simulink model "M_RALT"  (R2022a)
settings: Solver=ode4  StartTime=0.0  StopTime=100  FixedStep=0.01  RelTol=1e-3
PreLoadFcn:
  | listing = dir;
  | if (contains([listing .name], 'RALT')) && (contains([listing .name], 'MAP'))
  |     addpath('./RALT', './MAP', './DYN');
  |     addpath( genpath('./MAP') );
  | elseif (contains([listing .name], 'M_RALT.slx'))
  |     addpath('../RALT', '../MAP', '../DYN');
  |     addpath( genpath('../MAP') );
  | else
  | 
  | end
  | 
  | load('BUS_STRUCTURE_RALT.mat');
  | load('BUS_STRUCTURE_DYN.mat');
InitFcn:
  | listing = dir;
  | if (contains([listing .name], 'RALT')) && (contains([listing .name], 'MAP'))
  |     addpath('./RALT', './MAP', './DYN');
  |     addpath( genpath('./MAP') );
  | elseif (contains([listing .name], 'M_RALT.slx'))
  |     addpath('../RALT', '../MAP', '../DYN');
  |     addpath( genpath('../MAP') );
  | else
  | 
  | end
  | 
  | load('BUS_STRUCTURE_RALT.mat');
  | load('BUS_STRUCTURE_DYN.mat');
  | 
  | % Random number seed
  | if ~exist('ranNumSeed', 'var')
  |     ranNumSeed = 2034;
  | end
libraries: simulink x3
settings Model: Creator=ASCL  LastModifiedBy=ASCL
settings DataIOCC: SaveOutput=off  SignalLogging=off  DSMLogging=off  SaveTime=off  ReturnWorkspaceOutputs=off
settings OptimizationCC: BlockReduction=off  DefaultParameterBehavior=Inlined  UseDivisionForNetSlopeComputation=on  GainParamInheritBuiltInType=on  UseFloatMulNetSlope=on  ExpressionFolding=off  PassReuseOutputArgsAs=Individual arguments  ZeroExternalMemoryAtStartup=off  ZeroInternalMemoryAtStartup=off  EfficientFloat2IntCast=on  LifeSpan=inf  OptimizeBlockOrder=speed  DifferentSizesBufferReuse=on  EfficientTunableParamExpr=on
settings DebuggingCC: SignalInfNanChecking=warning  ReadBeforeWriteMsg=EnableAllAsError  WriteAfterWriteMsg=EnableAllAsError  WriteAfterReadMsg=EnableAllAsError  IntegerOverflowMsg=error  ParameterTunabilityLossMsg=error  UniqueDataStoreMsg=error  AssertControl=DisableAll  NonBusSignalsTreatedAsBus=error  SFInvalidInputDataAccessInChartInitDiag=error  SFTransitionOutsideNaturalParentDiag=error  SFUnreachableExecutionPathDiag=error  SFUndirectedBroadcastEventsDiag=error  IntegerSaturationMsg=error
settings HardwareCC: ProdBitPerPointer=32  ProdBitPerSizeT=32  ProdBitPerPtrDiffT=32  ProdLargestAtomicInteger=Long  ProdLargestAtomicFloat=Double  ProdEndianess=BigEndian  ProdWordSize=32  ProdLongLongMode=on  ProdHWDeviceType=Freescale->MPC83xx
settings ModelReferenceCC: ModelReferenceNumInstancesAllowed=Single
settings SFSimCC: SimCustomHeaderCode="#include \"MAP.h\""  SimUserSources=MAP.c  SimUserLibraries=WS2_32.LIB  CompileTimeRecursionLimit=0  EnableRuntimeRecursion=off  MATLABDynamicMemAlloc=off
settings RTWCC: SystemTargetFile=ert.tlc  TemplateMakefile=ert_default_tmf  GenerateReport=on  RTWUseSimCustomCode=on  CustomHeaderCode="#include \"MAP.h\""  CustomSource=MAP.c  CustomLibrary=WS2_32.LIB  BuildConfiguration=Faster Runs  IncludeHyperlinkInReport=on  LaunchReport=on  GenerateTraceInfo=on  GenerateTraceReport=on  GenerateTraceReportSl=on  GenerateTraceReportSf=on  GenerateTraceReportEml=on
settings CodeAppCC: ForceParamTrailComments=on  IgnoreCustomStorageClasses=off  OperatorAnnotations=on  SimulinkDataObjDesc=on  SFDataObjDesc=on  MATLABFcnDesc=on  InsertBlockDesc=on  StateflowObjectComments=on  MATLABSourceComments=on  EnableCustomComments=on  InlinedPrmAccess=Macros  ReqsInCode=on
settings ERTTargetCC: TargetLangStandard=C99 (ISO)  UtilityFuncGeneration=Shared location  GenerateSampleERTMain=on  IncludeMdlTerminateFcn=off  CombineSignalStateStructs=on  SupportAbsoluteTime=off  SupportNonFinite=off  SupportVariableSizeSignals=on  ParenthesesLevel=Standards  CastingMode=Standards  GenerateSharedConstants=off  InlinedParameterPlacement=NonHierarchical  ERTCustomFileTemplate=example_file_process.tlc  RateTransitionBlockCode=Function  PreserveIfCondition=on  ConvertIfToSwitch=off  EnableSignedLeftShifts=off  EnableSignedRightShifts=off

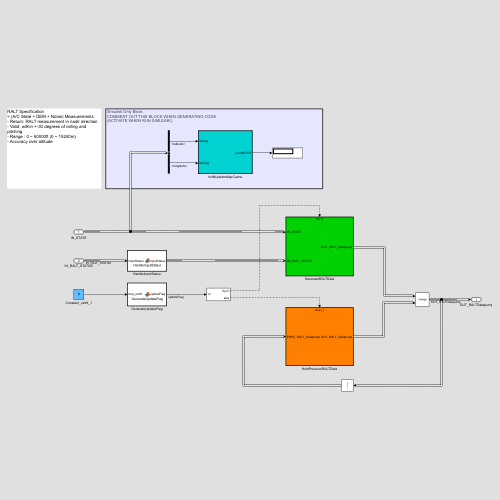
[thumbnail: Simulink's stored preview of the top-level diagram]
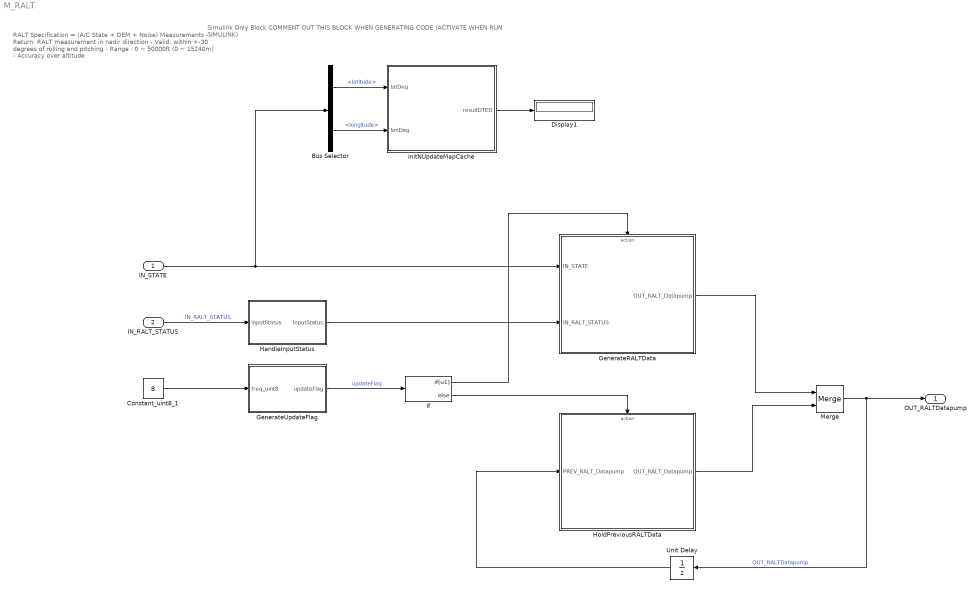
== system M_RALT ==
  note: Simulink Only Block
      | COMMENT OUT THIS BLOCK WHEN GENERATING CODE
      | (ACTIVATE WHEN RUN SIMULINK)
  note: RALT Specification
      | = (A/C State + DEM + Noise) Measurements
      | - Return: RALT measurement in nadir direction
      | - Valid: within +-30 degrees of rolling and pitching
      | - Range : 0 ~ 50000ft (0 ~ 15240m)
      | - Accuracy over altitude
  IN_STATE : Inport  OutDataTypeStr=Bus: BUS_DYN_STATE  Interpolate=off  BusOutputAsStruct=on
  IN_RALT_STATUS : Inport  Port=2  OutDataTypeStr=Bus: BUS_SENSOR_RALT_INPUTSTATUS  Interpolate=off  BusOutputAsStruct=on
  Bus Selector : BusSelector  OutputSignals=latitude,longitude
  Constant_uint8_1 : Constant  Value=8  OutDataTypeStr=uint8
  Display1 : Display
  GenerateRALTData : Subsystem  TreatAsAtomicUnit=on
  GenerateUpdateFlag : MATLAB Function  TreatAsAtomicUnit=on  SystemSampleTime=0.01
  HandleInputStatus : MATLAB Function  TreatAsAtomicUnit=on
  HoldPreviousRALTData : Subsystem  TreatAsAtomicUnit=on
  If : If  IfExpression=u1
  InitNUpdateMapCache : Subsystem  TreatAsAtomicUnit=on
  Merge : Merge
  Unit Delay : UnitDelay  SampleTime=-1  HasFrameUpgradeWarning=on
  OUT_RALTDatapump : Outport  OutDataTypeStr=Bus: BUS_SENSOR_RALT_DP  VectorParamsAs1DForOutWhenUnconnected=off  BusOutputAsStruct=on
  wires:
  InitNUpdateMapCache/1(resultDTED) -> Display1/1
  IN_STATE/1 -> GenerateRALTData/1(IN_STATE), Bus Selector/1
  IN_RALT_STATUS/1 -> HandleInputStatus/1("inputStatus ")  "IN_RALT_STATUS"
  HandleInputStatus/1(inputStatus) -> GenerateRALTData/2(IN_RALT_STATUS)
  Merge/1 -> Unit Delay/1, OUT_RALTDatapump/1  "OUT_RALTDatapump"
  GenerateRALTData/1(OUT_RALT_Datapump) -> Merge/1
  Constant_uint8_1/1 -> GenerateUpdateFlag/1(freq_uint8)
  GenerateUpdateFlag/1(updateFlag) -> If/1  "updateFlag"
  If/1 -> GenerateRALTData/Action
  HoldPreviousRALTData/1(OUT_RALT_Datapump) -> Merge/2
  If/2 -> HoldPreviousRALTData/Action
  Unit Delay/1 -> HoldPreviousRALTData/1(PREV_RALT_Datapump)
  Bus Selector/1 -> InitNUpdateMapCache/1(latDeg)  "<latitude>"
  Bus Selector/2 -> InitNUpdateMapCache/2(lonDeg)  "<longitude>"

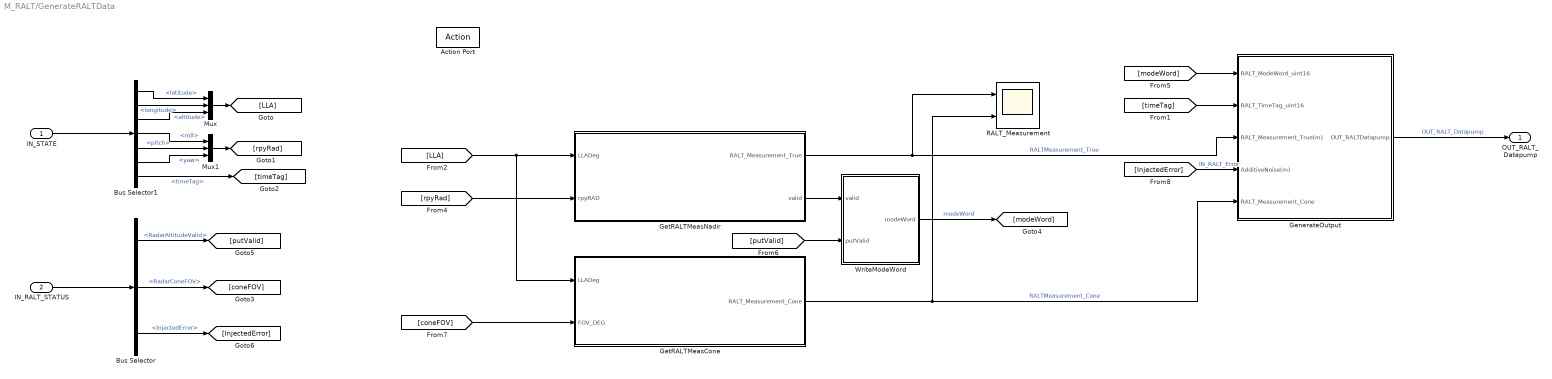
== system M_RALT/GenerateRALTData ==
  IN_STATE : Inport
  IN_RALT_STATUS : Inport  Port=2
  Action Port : ActionPort  ActionPortLabel=if(u1)
  Bus Selector : BusSelector  OutputSignals=RadarAltitudeValid,RadarConeFOV,InjectedError
  Bus Selector1 : BusSelector  OutputSignals=latitude,longitude,altitude,roll,pitch,yaw,timeTag
  GenerateOutput : Subsystem  TreatAsAtomicUnit=on
      settings: RTWSystemCode=Nonreusable function  RTWFcnNameOpts=Use subsystem name
  GetRALTMeasCone : Subsystem  TreatAsAtomicUnit=on
      settings: RTWSystemCode=Nonreusable function  RTWFcnNameOpts=Use subsystem name  FunctionInterfaceSpec=Allow arguments (Match graphical interface)
  GetRALTMeasNadir : Subsystem  TreatAsAtomicUnit=on
      settings: RTWSystemCode=Nonreusable function  RTWFcnNameOpts=Use subsystem name  FunctionInterfaceSpec=Allow arguments (Match graphical interface)
  Mux : Mux  Inputs=3
  Mux1 : Mux  Inputs=3
  RALT_Measurement : Scope  NumInputPorts=2
  WriteModeWord : MATLAB Function  TreatAsAtomicUnit=on  SystemSampleTime=0.01
  OUT_RALT_Datapump : Outport
  wires:
  [LLA] -> GetRALTMeasCone/1(LLADeg), GetRALTMeasNadir/1(LLADeg)
  GenerateOutput/1(OUT_RALTDatapump) -> OUT_RALT_Datapump/1  "OUT_RALT_Datapump"
  [rpyRad] -> GetRALTMeasNadir/2(rpyRAD)
  GetRALTMeasNadir/1(RALT_Measurement_True) -> RALT_Measurement/1, GenerateOutput/3(RALT_Measurement_True(m))  "RALTMeasurement_True"
  [modeWord] -> GenerateOutput/1(RALT_ModeWord_uint16)
  GetRALTMeasCone/1(RALT_Measurement_Cone) -> GenerateOutput/5(RALT_Measurement_Cone), RALT_Measurement/2  "RALTMeasurement_Cone"
  [putValid] -> WriteModeWord/2(putValid)
  [InjectedError] -> GenerateOutput/4(AdditiveNoise(m))  "IN_RALT_Error"
  GetRALTMeasNadir/2(valid) -> WriteModeWord/1(valid)
  WriteModeWord/1(modeWord) -> [modeWord]  "modeWord"
  Bus Selector1/4 -> Mux1/1  "<roll>"
  Bus Selector1/6 -> Mux1/3  "<yaw>"
  Bus Selector/1 -> [putValid]  "<RadarAltitudeValid>"
  Mux/1 -> [LLA]
  IN_RALT_STATUS/1 -> Bus Selector/1
  Bus Selector1/3 -> Mux/3  "<altitude>"
  IN_STATE/1 -> Bus Selector1/1
  Bus Selector1/5 -> Mux1/2  "<pitch>"
  Bus Selector1/1 -> Mux/1  "<latitude>"
  Bus Selector/3 -> [InjectedError]  "<InjectedError>"
  Bus Selector/2 -> [coneFOV]  "<RadarConeFOV>"
  Bus Selector1/2 -> Mux/2  "<longitude>"
  Mux1/1 -> [rpyRad]
  Bus Selector1/7 -> [timeTag]  "<timeTag>"
  [timeTag] -> GenerateOutput/2(RALT_TimeTag_uint16)
  [coneFOV] -> GetRALTMeasCone/2(FOV_DEG)

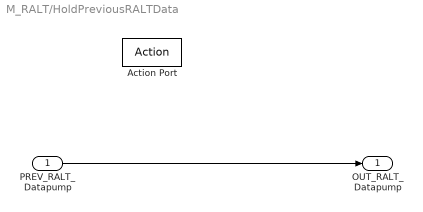
== system M_RALT/HoldPreviousRALTData ==
  PREV_RALT_Datapump : Inport
  Action Port : ActionPort  ActionPortLabel=else
  OUT_RALT_Datapump : Outport
  wires:
  PREV_RALT_Datapump/1 -> OUT_RALT_Datapump/1

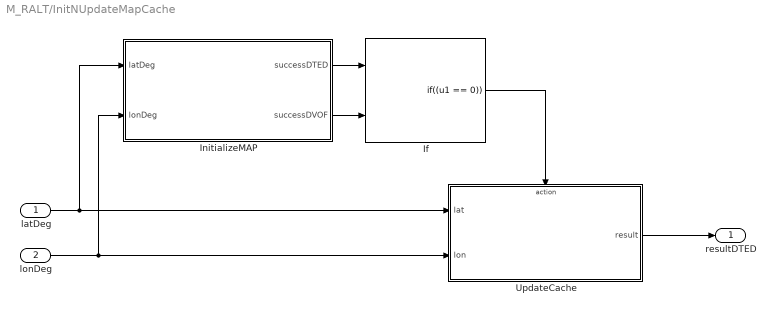
== system M_RALT/InitNUpdateMapCache ==
  latDeg : Inport  OutDataTypeStr=double
  lonDeg : Inport  Port=2  OutDataTypeStr=double
  If : If  NumInputs=2  IfExpression=(u1 == 0)  ShowElse=off
  InitializeMAP : MATLAB Function  TreatAsAtomicUnit=on
  UpdateCache : Subsystem  TreatAsAtomicUnit=on
  resultDTED : Outport  VectorParamsAs1DForOutWhenUnconnected=off
  wires:
  lonDeg/1 -> InitializeMAP/2(lonDeg), UpdateCache/2(lon)
  UpdateCache/1(result) -> resultDTED/1
  InitializeMAP/1(successDTED) -> If/1
  latDeg/1 -> InitializeMAP/1(latDeg), UpdateCache/1(lat)
  InitializeMAP/2(successDVOF) -> If/2
  If/1 -> UpdateCache/Action

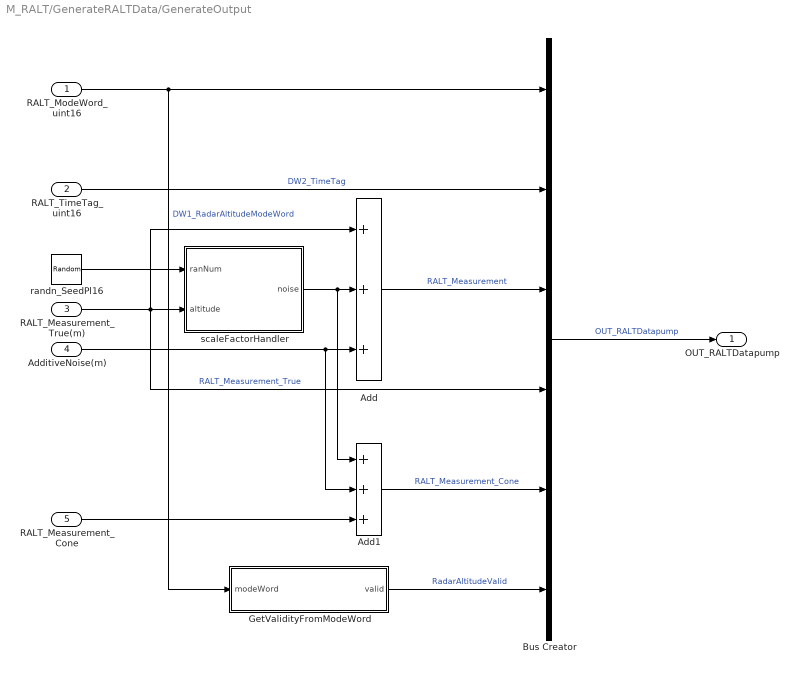
== system M_RALT/GenerateRALTData/GenerateOutput ==
  RALT_ModeWord_uint16 : Inport  OutDataTypeStr=fixdt('uint16', 'DataTypeOverride', 'Off')
  RALT_TimeTag_uint16 : Inport  Port=2  OutDataTypeStr=fixdt('uint16', 'DataTypeOverride', 'Off')
  RALT_Measurement_True(m) : Inport  Port=3
  AdditiveNoise(m) : Inport  Port=4
  RALT_Measurement_Cone : Inport  Port=5
  Add : Sum  Inputs=+++
  Add1 : Sum  Inputs=+++
  Bus Creator : BusCreator  Inputs=6  OutDataTypeStr=Bus: BUS_SENSOR_RALT_DP  NonVirtualBus=on
      settings: InheritFromInputs=off
  GetValidityFromModeWord : MATLAB Function  TreatAsAtomicUnit=on
  randn_SeedPl16 : RandomNumber  Seed=(ranNumSeed+16)  SampleTime=0.01
  scaleFactorHandler : MATLAB Function  TreatAsAtomicUnit=on
  OUT_RALTDatapump : Outport  OutDataTypeStr=Bus: BUS_SENSOR_RALT_DP
  wires:
  RALT_Measurement_True(m)/1 -> Bus Creator/4, Add/1, scaleFactorHandler/2(altitude)  "RALT_Measurement_True"
  AdditiveNoise(m)/1 -> Add1/2, Add/3
  scaleFactorHandler/1(noise) -> Add1/1, Add/2
  randn_SeedPl16/1 -> scaleFactorHandler/1(ranNum)
  RALT_TimeTag_uint16/1 -> Bus Creator/2  "DW2_TimeTag"
  Bus Creator/1 -> OUT_RALTDatapump/1  "OUT_RALTDatapump"
  RALT_ModeWord_uint16/1 -> GetValidityFromModeWord/1(modeWord), Bus Creator/1  "DW1_RadarAltitudeModeWord"
  Add/1 -> Bus Creator/3  "RALT_Measurement"
  Add1/1 -> Bus Creator/5  "RALT_Measurement_Cone"
  RALT_Measurement_Cone/1 -> Add1/3
  GetValidityFromModeWord/1(valid) -> Bus Creator/6  "RadarAltitudeValid"

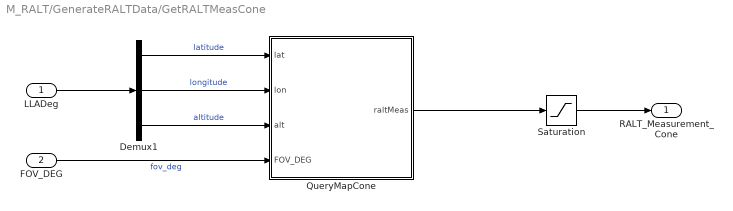
== system M_RALT/GenerateRALTData/GetRALTMeasCone ==
  LLADeg : Inport
  FOV_DEG : Inport  Port=2
  Demux1 : Demux  Outputs=3
  QueryMapCone : Subsystem
  Saturation : Saturate  UpperLimit=15240  LowerLimit=0
  RALT_Measurement_Cone : Outport
  wires:
  Saturation/1 -> RALT_Measurement_Cone/1
  QueryMapCone/1(raltMeas) -> Saturation/1
  Demux1/3 -> QueryMapCone/3(alt)  "altitude"
  Demux1/1 -> QueryMapCone/1(lat)  "latitude"
  Demux1/2 -> QueryMapCone/2(lon)  "longitude"
  LLADeg/1 -> Demux1/1
  FOV_DEG/1 -> QueryMapCone/4(FOV_DEG)  "fov_deg"

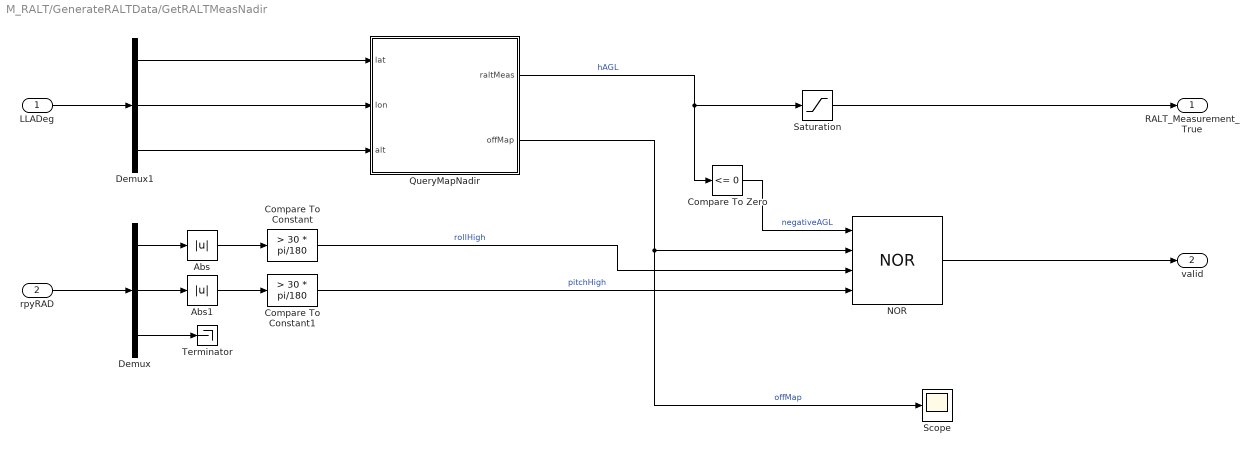
== system M_RALT/GenerateRALTData/GetRALTMeasNadir ==
  LLADeg : Inport
  rpyRAD : Inport  Port=2
  Abs : Abs  SaturateOnIntegerOverflow=off
  Abs1 : Abs  SaturateOnIntegerOverflow=off
  Compare To Constant : simulink/Logic and Bit Operations/Compare To Constant  relop=>  const=30 * pi/180  OutDataTypeStr=boolean
  Compare To Constant1 : simulink/Logic and Bit Operations/Compare To Constant  relop=>  const=30 * pi/180  OutDataTypeStr=boolean
  Compare To Zero : simulink/Logic and Bit Operations/Compare To Zero  relop=<=  OutDataTypeStr=boolean
  Demux : Demux  Outputs=3
  Demux1 : Demux  Outputs=3
  NOR : Logic  Operator=NOR  Inputs=4  AllPortsSameDT=off  OutDataTypeStr=boolean
  QueryMapNadir : Subsystem
  Saturation : Saturate  UpperLimit=15240  LowerLimit=0
  Scope : Scope
  Terminator : Terminator
  RALT_Measurement_True : Outport
  valid : Outport  Port=2
  wires:
  rpyRAD/1 -> Demux/1
  LLADeg/1 -> Demux1/1
  Demux/3 -> Terminator/1
  Demux/1 -> Abs/1
  Demux/2 -> Abs1/1
  Abs/1 -> Compare To Constant/1
  Abs1/1 -> Compare To Constant1/1
  Demux1/2 -> QueryMapNadir/2(lon)
  Demux1/1 -> QueryMapNadir/1(lat)
  Demux1/3 -> QueryMapNadir/3(alt)
  QueryMapNadir/1(raltMeas) -> Compare To Zero/1, Saturation/1  "hAGL"
  Compare To Constant/1 -> NOR/3  "rollHigh"
  Compare To Constant1/1 -> NOR/4  "pitchHigh"
  Compare To Zero/1 -> NOR/1  "negativeAGL"
  Saturation/1 -> RALT_Measurement_True/1
  QueryMapNadir/2(offMap) -> Scope/1, NOR/2  "offMap"
  NOR/1 -> valid/1

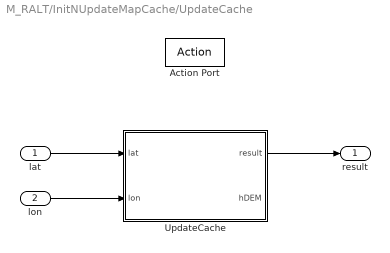
== system M_RALT/InitNUpdateMapCache/UpdateCache ==
  lat : Inport
  lon : Inport  Port=2
  Action Port : ActionPort  ActionPortLabel=if((u1 == 0))
  UpdateCache : MATLAB Function  TreatAsAtomicUnit=on
  result : Outport  VectorParamsAs1DForOutWhenUnconnected=off
  wires:
  UpdateCache/1(result) -> result/1
  lat/1 -> UpdateCache/1(lat)
  lon/1 -> UpdateCache/2(lon)

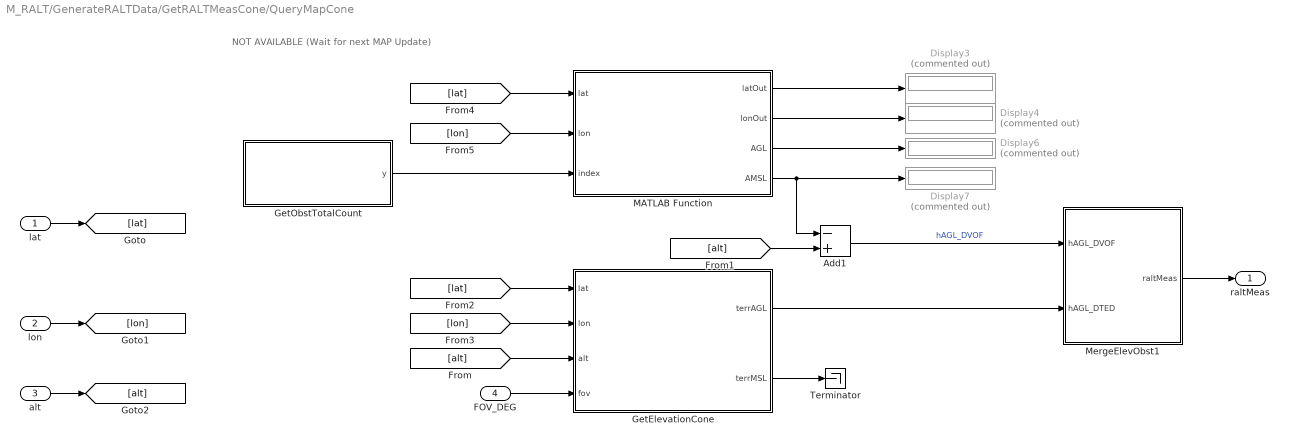
== system M_RALT/GenerateRALTData/GetRALTMeasCone/QueryMapCone ==
  note: NOT AVAILABLE (Wait for next MAP Update)
  lat : Inport
  lon : Inport  Port=2
  alt : Inport  Port=3
  FOV_DEG : Inport  Port=4
  Add1 : Sum  Inputs=-+
  Display{3..4,6..7} (4 alike) : Display  Commented=on
  GetElevationCone : MATLAB Function  TreatAsAtomicUnit=on
  GetObstTotalCount : MATLAB Function  TreatAsAtomicUnit=on
  MATLAB Function : MATLAB Function  TreatAsAtomicUnit=on
  MergeElevObst1 : MATLAB Function  TreatAsAtomicUnit=on
  Terminator : Terminator
  raltMeas : Outport  VectorParamsAs1DForOutWhenUnconnected=off
  wires:
  [lat] -> GetElevationCone/1(lat)
  [lon] -> MATLAB Function/2(lon)
  [lat] -> MATLAB Function/1(lat)
  MATLAB Function/3(AGL) -> Display6/1
  lat/1 -> [lat]
  MATLAB Function/2(lonOut) -> Display4/1
  lon/1 -> [lon]
  MATLAB Function/1(latOut) -> Display3/1
  MATLAB Function/4(AMSL) -> Display7/1, Add1/1
  GetElevationCone/1(terrAGL) -> MergeElevObst1/2(hAGL_DTED)
  GetObstTotalCount/1(y) -> MATLAB Function/3(index)
  [lon] -> GetElevationCone/2(lon)
  alt/1 -> [alt]
  [alt] -> GetElevationCone/3(alt)
  GetElevationCone/2(terrMSL) -> Terminator/1
  Add1/1 -> MergeElevObst1/1(hAGL_DVOF)  "hAGL_DVOF"
  [alt] -> Add1/2
  MergeElevObst1/1(raltMeas) -> raltMeas/1
  FOV_DEG/1 -> GetElevationCone/4(fov)

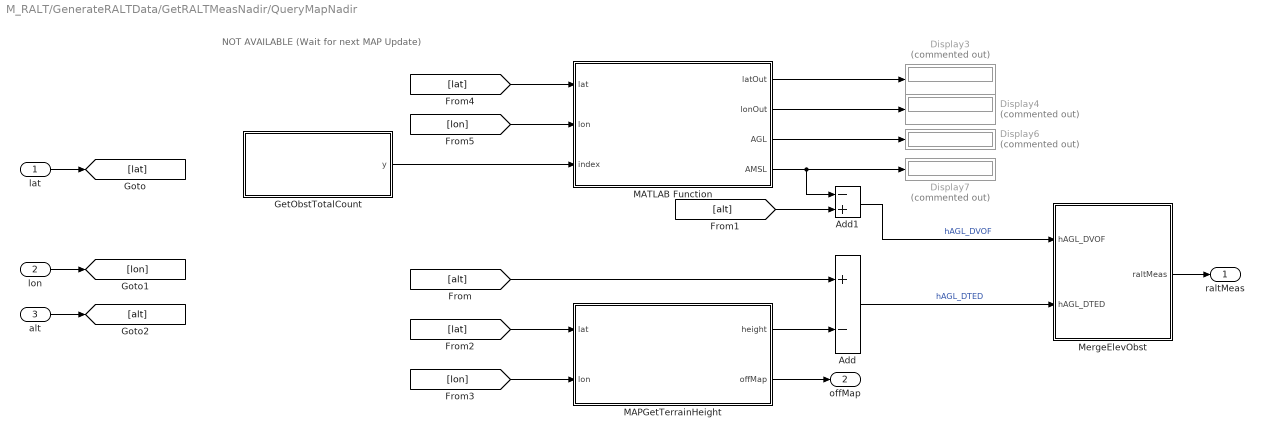
== system M_RALT/GenerateRALTData/GetRALTMeasNadir/QueryMapNadir ==
  note: NOT AVAILABLE (Wait for next MAP Update)
  lat : Inport
  lon : Inport  Port=2
  alt : Inport  Port=3
  Add : Sum  Inputs=+-
  Add1 : Sum  Inputs=-+
  Display{3..4,6..7} (4 alike) : Display  Commented=on
  GetObstTotalCount : MATLAB Function  TreatAsAtomicUnit=on
  MAPGetTerrainHeight : MATLAB Function  TreatAsAtomicUnit=on
  MATLAB Function : MATLAB Function  TreatAsAtomicUnit=on
  MergeElevObst : MATLAB Function  TreatAsAtomicUnit=on
  raltMeas : Outport  VectorParamsAs1DForOutWhenUnconnected=off
  offMap : Outport  Port=2
  wires:
  [lat] -> MAPGetTerrainHeight/1(lat)
  [lon] -> MATLAB Function/2(lon)
  [lat] -> MATLAB Function/1(lat)
  MATLAB Function/3(AGL) -> Display6/1
  lat/1 -> [lat]
  MATLAB Function/2(lonOut) -> Display4/1
  lon/1 -> [lon]
  MATLAB Function/1(latOut) -> Display3/1
  MATLAB Function/4(AMSL) -> Display7/1, Add1/1
  GetObstTotalCount/1(y) -> MATLAB Function/3(index)
  [lon] -> MAPGetTerrainHeight/2(lon)
  MAPGetTerrainHeight/1(height) -> Add/2
  alt/1 -> [alt]
  Add/1 -> MergeElevObst/2(hAGL_DTED)  "hAGL_DTED"
  [alt] -> Add/1
  Add1/1 -> MergeElevObst/1(hAGL_DVOF)  "hAGL_DVOF"
  [alt] -> Add1/2
  MergeElevObst/1(raltMeas) -> raltMeas/1
  MAPGetTerrainHeight/2(offMap) -> offMap/1

== matlab function M_RALT/GenerateRALTData/GetRALTMeasNadir/QueryMapNadir/GetObstTotalCount ==
  data: y output
function y = GetObstTotalCount()

count = -2;

% count = coder.ceval('GetObstTotalCount');

y = count;

== matlab function M_RALT/GenerateRALTData/GetRALTMeasNadir/QueryMapNadir/MAPGetTerrainHeight ==
  data: lat input; height output; lon input; offMap output
function [height, offMap] = MAPGetTerrainHeight(lat, lon)
%MAPGetTerrainHeight

% Initialize
height = 0.0;
offMap = false;

height = coder.ceval('MAPGetTerrainHeight', lat, lon);

if (height < -0.5)
    offMap = true;
else
end

== matlab function M_RALT/GenerateRALTData/GetRALTMeasNadir/QueryMapNadir/MATLAB Function ==
  data: lat input; lon input; index input; latOut output; lonOut output; AGL output; AMSL output
function [latOut, lonOut, AGL, AMSL] = GetObstacleInfo(lat, lon, index)

% Constant
DEG2RAD = 0.017453292519943;
EARTH_RADIUS = 6378137;

% Initialize
latOut  = 0.0;
lonOut  = 0.0;
AGL     = 0.0;
AMSL    = 0.0;
AMSLI   = 0.0;
dist    = 0.0;


% if index>=0
%     for i=0:index-1
%         latOut = coder.ceval('GetObstacleInfo', lat, lon, i, 1);
%         lonOut = coder.ceval('GetObstacleInfo', lat, lon, i, 2);
%         AGL    = coder.ceval('GetObstacleInfo', lat, lon, i, 3);
% 
%         % Roughly calculate distance
%         dist=sqrt(((lat-latOut)*DEG2RAD*EARTH_RADIUS)^2+((lon-lonOut)*DEG2RAD*EARTH_RADIUS)^2);
% 
%         if (dist < AGL)
%             AMSLI = coder.ceval('GetObstacleInfo', lat, lon, i, 4);
%             if AMSLI > AMSL
%                 AMSL = AMSLI;
%             end
%         end
%     end
end

== matlab function M_RALT/GenerateRALTData/GetRALTMeasNadir/QueryMapNadir/MergeElevObst ==
  data: hAGL_DVOF input; raltMeas output; hAGL_DTED input
function raltMeas = MergeElevObst(hAGL_DVOF, hAGL_DTED)
%MergeElevObst
raltMeas = hAGL_DTED;

if hAGL_DVOF < hAGL_DTED
    raltMeas = hAGL_DVOF;
end

== matlab function M_RALT/GenerateRALTData/WriteModeWord ==
  data: valid input; modeWord output; putValid input
function modeWord = WriteModeWord(valid, putValid)
%WriteModeWord
persistent count
if isempty(count)
    count = uint8(0);
end

% Intiailize
modeWord = uint16(0);

if (valid) && (putValid) && (count < uint8(4))
    % Radar altitude valid
    modeWord = uint16(0b0000000000000110);
    count = count + uint8(1);
elseif (valid) && (putValid) && (count >= uint8(4))
    % Radar altitude valid & Radar altitude rate valid
    modeWord = uint16(0b0000000000001110);
else
    % Not valid
    modeWord = uint16(0b0000000000000010);
    count = uint8(0);
end

== matlab function M_RALT/GenerateUpdateFlag ==
  settings: updateMethod=DISCRETE  sampleTime=0.01
  data: updateFlag output boolean; freq_uint8 input uint8
function updateFlag = GenerateUpdateFlag(freq_uint8)
%GenerateUpdateFlag RALT 데이터 갱신 플래그 생성
% Input
% - freq_uint8  1 = update data at every simulation step
%               25 = update data at every 25 simulation steps
%               Accepts  (8bit unsigned integer=uint8) only
% Output
% - updateFlag  True/False
persistent cnt

assert (isa(freq_uint8, 'uint8'))

if isempty(cnt)
    cnt = uint8(0);
end

% Initialize
updateFlag = false;

if mod(cnt, freq_uint8) == uint8(0)
    updateFlag = true;
    cnt = uint8(1);
else
    updateFlag = false;
    cnt = cnt + uint8(1);
end

end

== matlab function M_RALT/InitNUpdateMapCache/InitializeMAP ==
  data: successDTED output; successDVOF output; latDeg input; lonDeg input
function [successDTED, successDVOF] = InitializeMAP(latDeg, lonDeg)
%InitializeMAP

% Persistent variable
persistent firstRun
if isempty(firstRun)
    firstRun = true;
end

% Initialize output
flagDTED = int32(1);
flagDVOF = int32(1);
successDTED = int32(1);
successDVOF = int32(1);
hDEM = 0.0;

if firstRun
    % Path of DTED data
    pathDTED = 'C:\Users\ASCL\Documents\GitHub\DTNS\MAP\MAP_DB';

    % Length of DETD data path
    strLenDTED = int32(strlength(pathDTED));
    
    hDEM = coder.ceval('MAPGetTerrainHeight', latDeg, lonDeg);
    if IsNear(hDEM, -1.0)
        % Call [ InitialMap ] : 맵 폴더 위치 설정
        flagDTED = coder.ceval('InitialMap', pathDTED, strLenDTED );
        successDTED = flagDTED;
        if (~successDTED)
            firstRun = false;
        end
    else
        successDTED = int32(0);
        firstRun = false;       
    end
else
    successDTED = int32(0);
    successDVOF = int32(0);
end

== matlab function M_RALT/HandleInputStatus ==
  data: inputStatus input Bus: BUS_SENSOR_RALT_INPUTSTATUS; inputStatus output
function inputStatus = HandleInputStatus(inputStatus)

if(inputStatus.InputActivated)
    
else
    inputStatus.RadarAltitudeValid = true;
    inputStatus.RadarConeFOV = 30;
end

== matlab function M_RALT/GenerateRALTData/GenerateOutput/GetValidityFromModeWord ==
  data: modeWord input; valid output
function valid = GetValidityFromModeWord(modeWord)
%GetValidityFromModeWord

valid = logical( bitget(modeWord, 3) );

== matlab function M_RALT/InitNUpdateMapCache/UpdateCache/UpdateCache ==
  data: result output; lat input; lon input; hDEM output
function [result, hDEM] = UpdateCache(lat, lon)
%UpdateCache

% Persistent variables
persistent latPrev lonPrev
if isempty(latPrev)
    latPrev = 0.0;
end
if isempty(lonPrev)
    lonPrev = 0.0;
end

hDEM = 0.0;

% Initialize output
result = int32(1);

if ( abs(lat - latPrev) > 0.05 ) || ( abs(lon - lonPrev) > 0.05)
    fprintf("RALT UpdateCache - lat: %3.7f, lon: %3.7f, latPrev: %3.7f, lonPrev: %3.7f \r\n", lat, lon, latPrev, lonPrev);

    result = coder.ceval('UpdateCache', lat, lon);
    hDEM = coder.ceval('MAPGetTerrainHeight', lat, lon);

    if result == 0
        latPrev = lat;
        lonPrev = lon;
    end
else
    
end

== matlab function M_RALT/GenerateRALTData/GenerateOutput/scaleFactorHandler ==
  data: ranNum input; noise output; altitude input
function noise = scaleFactorHandler(ranNum, altitude)

if altitude <= 30.48
    noise = 0.6096 * (1/3);
elseif (altitude > 30.48) && (altitude <= 1524)
    noise = altitude * (2/100) * (1/3);
elseif (altitude > 1524) && (altitude <= 3048)
    noise = 30.48 * (1/3);
elseif (altitude > 3048)
    noise = altitude * (1/100) * (1/3);
else
    noise = 0.6096 * (1/3);
end

noise = ranNum * noise;

== matlab function M_RALT/GenerateRALTData/GetRALTMeasCone/QueryMapCone/GetElevationCone ==
  data: lat input; terrAGL output; lon input; alt input; terrMSL output; fov input
function [terrAGL, terrMSL] = GetElevationCone(lat, lon, alt, fov)
%GetElevationCone
% Find first return (nearest)

% Intiailize
slantR = 0.0;
terrNadir = 0.0;
terrTemp = 0.0;
terrMSL = 0.0;

% Nadir point
terrNadir = coder.ceval('MAPGetTerrainHeight', lat, lon);
terrAGL = alt - terrNadir;

if (terrAGL <= 0)
    terrAGL = 0.0;
    return
else

    % FOV/2 saturated on [0, 30]
    fovUsed = max(0, min(fov/2, 30));
    
    % Horizontal length of FOV saturated on [0, 1524*tand(fovUsed)]
    L = tand(fovUsed) * terrAGL;
    L = max(0, min(L, tand(fovUsed)*1524));

    % Length of a degree
    [latLength, lonLength] = getLengthOfADegree(lat, terrNadir);

    for cc = 1:3
        
        % Horizontal length of current iteration
        curL = (cc/3) * L;
        
        for rr = 1:8

            % Query point
            curLat = lat + curL / latLength * sind(45*rr);
            curLon = lon + curL / lonLength * cosd(45*rr);
            
            terrTemp = coder.ceval('MAPGetTerrainHeight', curLat, curLon);
            terrAGLTemp = alt - terrTemp;

            if terrAGLTemp < 0
                slantR = curL;
            else
                slantR = sqrt(curL^2 + terrAGLTemp^2);
            end

            if (slantR < terrAGL)
                terrAGL = slantR;
            end
        end
    end
end

terrMSL = alt - terrAGL;

end

function [latLength, lonLength] = getLengthOfADegree(lat, h)
%GETLENGTHOFADEGREE
% Calculate the length of one degree of both latitude and longitude
% for a specified latitude and height
%
% == Inputs =========
% lat               - Latitude [deg]
% h                 - Height [m]
% 
% == Outputs ========
% latLength         - Length of 1 deg of latitude on the ref. spheroid [m]
% lonLength         - Length of 1 deg of longitude on the ref. spheroid [m]
% ===================

% WGS84 Parameters
eRadius = 6378137.0;
eEccen = 0.08181919;

% Radius of curvature in prime vertical
nE = eRadius / sqrt( 1 - (eEccen^2*(sind(lat))^2) );
% Meridian Radius of Curavature
mE = eRadius * (1 - eEccen^2) / (1 - eEccen^2*(sind(lat))^2)^(1.5);

lonLength = (nE + h) * cosd(lat) * (pi/180);
latLength = (mE + h) * (pi/180);

end

== matlab function M_RALT/GenerateRALTData/GetRALTMeasCone/QueryMapCone/GetObstTotalCount ==
  data: y output
function y = GetObstTotalCount()

count = -2;

% count = coder.ceval('GetObstTotalCount');

y = count;

== matlab function M_RALT/GenerateRALTData/GetRALTMeasCone/QueryMapCone/MATLAB Function ==
  data: lat input; lon input; index input; latOut output; lonOut output; AGL output; AMSL output
function [latOut, lonOut, AGL, AMSL] = GetObstacleInfo(lat, lon, index)

% Constant
DEG2RAD = 0.017453292519943;
EARTH_RADIUS = 6378137;

% Initialize
latOut  = 0.0;
lonOut  = 0.0;
AGL     = 0.0;
AMSL    = 0.0;
AMSLI   = 0.0;
dist    = 0.0;


% if index>=0
%     for i=0:index-1
%         latOut = coder.ceval('GetObstacleInfo', lat, lon, i, 1);
%         lonOut = coder.ceval('GetObstacleInfo', lat, lon, i, 2);
%         AGL    = coder.ceval('GetObstacleInfo', lat, lon, i, 3);
% 
%         % Roughly calculate distance
%         dist=sqrt(((lat-latOut)*DEG2RAD*EARTH_RADIUS)^2+((lon-lonOut)*DEG2RAD*EARTH_RADIUS)^2);
% 
%         if (dist < AGL)
%             AMSLI = coder.ceval('GetObstacleInfo', lat, lon, i, 4);
%             if AMSLI > AMSL
%                 AMSL = AMSLI;
%             end
%         end
%     end
% else
end

== matlab function M_RALT/GenerateRALTData/GetRALTMeasCone/QueryMapCone/MergeElevObst1 ==
  data: hAGL_DVOF input; raltMeas output; hAGL_DTED input
function raltMeas = MergeElevObst(hAGL_DVOF, hAGL_DTED)
%MergeElevObst
raltMeas = hAGL_DTED;

if hAGL_DVOF < hAGL_DTED
    raltMeas = hAGL_DVOF;
end
